simulink model "cart_pend"  (Simulink 7.1)
settings: Solver=ode23  StartTime=0.0  StopTime=5  RelTol=1e-6
values from neighbouring files (symbols this model uses):
  g = 9.81    [MPCsimulink.m]    (also in assignment4.m; pend_init.m; setupOptimization.m)
  g1 = c2d(tf([1 0],[tcAngleVel 1]),h,'tustin')    [assignment4.m]    (also in assignment5.m; pend_init.m)
  g2 = c2d(tf(1,[tcAngle 1]),h,'tustin')    [assignment4.m]    (also in assignment5.m; pend_init.m)
  g3 = c2d(tf(1),h)    [assignment1.m]    (also in assignment3.m = c2d(tf(1,[tcAcc 1]),h,'tustin'); assignment4.m = c2d(tf(1,[tcAcc 1]),h,'tustin'); assignment5.m = c2d(tf(1,[tcAcc 1]),h,'tustin'); pend_init.m = c2d(tf(1,[tcAcc 1]),h,'tustin'))
  h = uIn(5*N+10)    [MPCsimulink.m]    (also in assignment1.m = 0.001; pend_init.m = 0.01)
  initPendValue = [0;0]    [assignment3.m]    (also in assignment4.m; pend_init.m)
  initPosError = 0    [assignment1.m]    (also in assignment3.m; assignment4.m; assignment5.m; pend_init.m)
  l = 0.345    [MPCsimulink.m]    (also in assignment4.m; loaddym.m = fgetl(fid); pend_init.m)
  N = uIn(end)    [MPCsimulink.m]    (also in assignment3.m = -1; assignment5.m = %---------------------------------------------------------; setupOptimization.m = length(theta))
  p0 = -1.5    [assignment1.m]    (also in assignment5.m = -0.8)
  Q = sparse(Q)    [MPCsimulink.m]    (also in assignment3.m = 0; assignment4.m = [  R =; assignment5.m = [  R =)
  R = 0    [assignment3.m]
libraries: simulink x1
settings Model: Creator=pontusg  LastModifiedBy=pontusg  ExtModeAutoUpdateStatusClock=off
settings DataIOCC: Refine=10
settings DebuggingCC: SaveWithParameterizedLinksMsg=none
settings GRTTargetCC: TargetFcnLib=ansi_tfl_tmw.mat

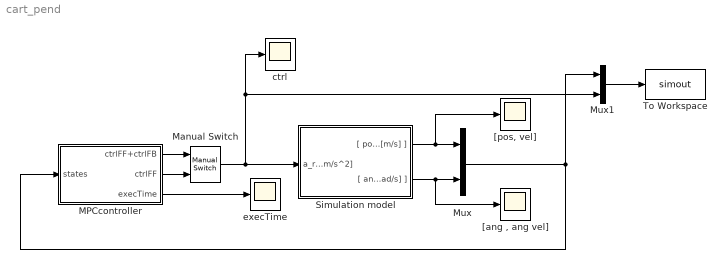
== system cart_pend ==
  MPCcontroller : Subsystem
  Manual Switch : simulink/Signal Routing/Manual Switch  SystemSampleTime=-1  sw=1  action=0  varsize=off
  Mux : Mux  Inputs=2
  Mux1 : Mux  Inputs=2
  Simulation model : Subsystem
  To Workspace : ToWorkspace  VariableName=simout  SampleTime=-1  SaveFormat=Structure With Time
  "[ang , ang vel]" : Scope
      settings: TimeRange=10  YMin=-0.5  YMax=3.25
  "[pos, vel]" : Scope
      settings: TimeRange=6  YMin=-0.0575  YMax=-0.0075
  ctrl : Scope
      settings: TimeRange=10  YMin=-0.5  YMax=3.25  SaveName=ScopeData2
  execTime : Scope
      settings: TimeRange=10  YMin=-0.5  YMax=3.25  SaveName=ScopeData3
  wires:
  Simulation model/1("[ pos [m] , vel [m/s] ]") -> Mux/1, "[pos, vel]"/1
  Mux/1 -> Mux1/1, MPCcontroller/1(states)
  Mux1/1 -> To Workspace/1
  Simulation model/2("[ ang [rad] , angVel [rad/s] ]") -> Mux/2, "[ang , ang vel]"/1
  MPCcontroller/1(ctrlFF+ctrlFB) -> Manual Switch/1
  MPCcontroller/2(ctrlFF) -> Manual Switch/2
  Manual Switch/1 -> ctrl/1, Mux1/2, Simulation model/1(a_ref [m/s^2])
  MPCcontroller/3(execTime) -> execTime/1

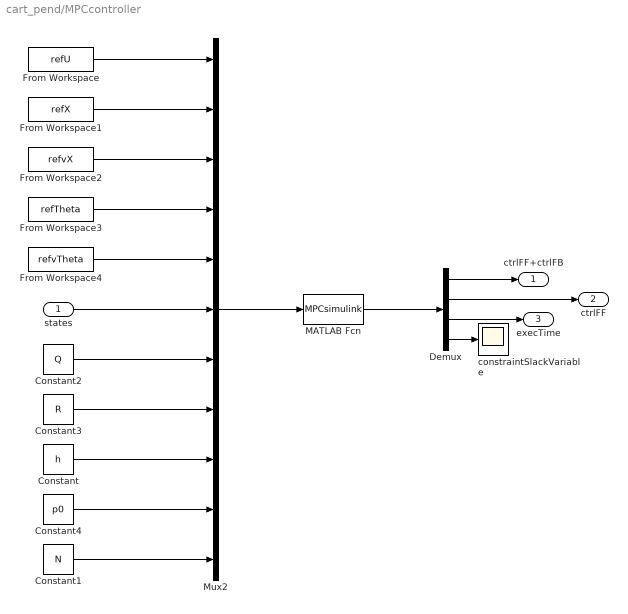
== system cart_pend/MPCcontroller ==
  states : Inport  OutDataType=sfix(16)  OutScaling=2^0
  Constant : Constant  Value=h  OutDataType=sfix(16)  OutScaling=2^0  SampleTime=h
  Constant1 : Constant  Value=N  OutDataType=sfix(16)  OutScaling=2^0  SampleTime=h
  Constant2 : Constant  Value=Q  OutDataType=sfix(16)  OutScaling=2^0  SampleTime=h
  Constant3 : Constant  Value=R  OutDataType=sfix(16)  OutScaling=2^0  SampleTime=h
  Constant4 : Constant  Value=p0  OutDataType=sfix(16)  OutScaling=2^0  SampleTime=h
  Demux : Demux  Outputs=[1 1 1 1]
  From Workspace : FromWorkspace  VariableName=refU  SampleTime=h  Interpolate=off  OutputAfterFinalValue=Holding final value
  From Workspace1 : FromWorkspace  VariableName=refX  SampleTime=h  Interpolate=off  OutputAfterFinalValue=Holding final value
  From Workspace2 : FromWorkspace  VariableName=refvX  SampleTime=h  Interpolate=off  OutputAfterFinalValue=Holding final value
  From Workspace3 : FromWorkspace  VariableName=refTheta  SampleTime=h  Interpolate=off  OutputAfterFinalValue=Holding final value
  From Workspace4 : FromWorkspace  VariableName=refvTheta  SampleTime=h  Interpolate=off  OutputAfterFinalValue=Holding final value
  MATLAB Fcn : MATLABFcn  MATLABFcn=MPCsimulink  OutputDimensions=4
  Mux2 : Mux  Inputs=11
  constraintSlackVariable : Scope
      settings: TimeRange=8.378423004623279  YMin=0.004183789062500001  YMax=0.004352539062500001  SaveName=ScopeData6
  ctrlFF+ctrlFB : Outport  OutDataType=sfix(16)  OutScaling=2^0
  ctrlFF : Outport  Port=2  OutDataType=sfix(16)  OutScaling=2^0
  execTime : Outport  Port=3  OutDataType=sfix(16)  OutScaling=2^0
  wires:
  From Workspace/1 -> Mux2/1
  From Workspace1/1 -> Mux2/2
  From Workspace2/1 -> Mux2/3
  From Workspace3/1 -> Mux2/4
  From Workspace4/1 -> Mux2/5
  Mux2/1 -> MATLAB Fcn/1
  Demux/1 -> ctrlFF+ctrlFB/1
  Demux/2 -> ctrlFF/1
  MATLAB Fcn/1 -> Demux/1
  states/1 -> Mux2/6
  Constant2/1 -> Mux2/7
  Constant3/1 -> Mux2/8
  Constant/1 -> Mux2/9
  Demux/3 -> execTime/1
  Demux/4 -> constraintSlackVariable/1
  Constant4/1 -> Mux2/10
  Constant1/1 -> Mux2/11

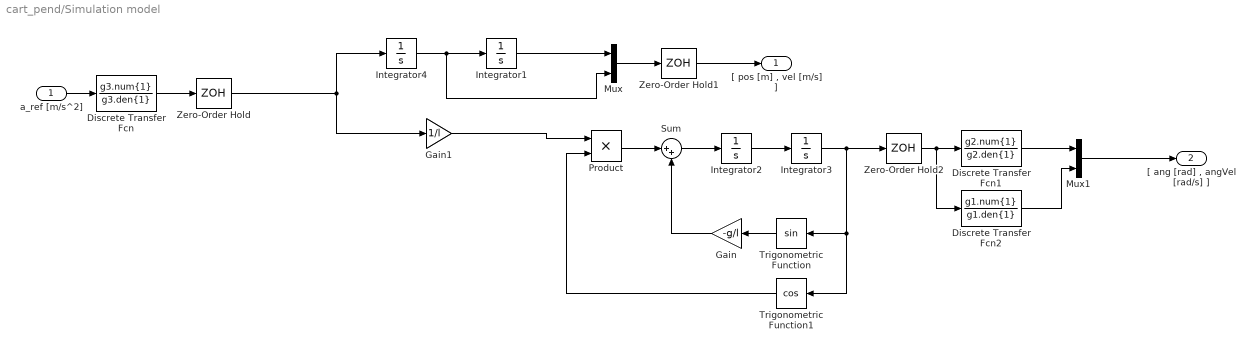
== system cart_pend/Simulation model ==
  a_ref [m/s^2] : Inport  OutDataType=sfix(16)  OutScaling=2^0
  Discrete Transfer Fcn : DiscreteTransferFcn  Numerator=g3.num{1}  Denominator=g3.den{1}  SampleTime=h
  Discrete Transfer Fcn1 : DiscreteTransferFcn  Numerator=g2.num{1}  Denominator=g2.den{1}  SampleTime=h
  Discrete Transfer Fcn2 : DiscreteTransferFcn  Numerator=g1.num{1}  Denominator=g1.den{1}  SampleTime=h
  Gain : Gain  Orientation=left  Gain=-g/l  ParameterDataType=sfix(16)  ParameterScaling=2^0  OutDataType=sfix(16)  OutScaling=2^0
  Gain1 : Gain  Gain=1/l  ParameterDataType=sfix(16)  ParameterScaling=2^0  OutDataType=sfix(16)  OutScaling=2^0
  Integrator1 : Integrator  InitialCondition=p0+initPosError
  Integrator2 : Integrator  InitialCondition=initPendValue(2)
  Integrator3 : Integrator  InitialCondition=initPendValue(1)
  Integrator4 : Integrator
  Mux : Mux  Inputs=2
  Mux1 : Mux  Inputs=2
  Product : Product  OutDataType=sfix(16)  OutScaling=2^0  RndMeth=Zero
  Sum : Sum  Inputs=|++  OutDataType=sfix(16)  OutScaling=2^0
  Trigonometric Function : Trigonometry  Orientation=left
  Trigonometric Function1 : Trigonometry  Orientation=left  Operator=cos
  Zero-Order Hold : ZeroOrderHold  SampleTime=h
  Zero-Order Hold1 : ZeroOrderHold  SampleTime=h
  Zero-Order Hold2 : ZeroOrderHold  SampleTime=h
  "[ pos [m] , vel [m/s] ]" : Outport  OutDataType=sfix(16)  OutScaling=2^0
  "[ ang [rad] , angVel [rad/s] ]" : Outport  Port=2  OutDataType=sfix(16)  OutScaling=2^0
  wires:
  Zero-Order Hold1/1 -> "[ pos [m] , vel [m/s] ]"/1
  Zero-Order Hold/1 -> Gain1/1, Integrator4/1
  Integrator4/1 -> Integrator1/1, Mux/2
  Integrator1/1 -> Mux/1
  Integrator2/1 -> Integrator3/1
  Integrator3/1 -> Trigonometric Function/1, Trigonometric Function1/1, Zero-Order Hold2/1
  Sum/1 -> Integrator2/1
  Mux/1 -> Zero-Order Hold1/1
  Mux1/1 -> "[ ang [rad] , angVel [rad/s] ]"/1
  a_ref [m/s^2]/1 -> Discrete Transfer Fcn/1
  Gain1/1 -> Product/1
  Product/1 -> Sum/1
  Trigonometric Function1/1 -> Product/2
  Trigonometric Function/1 -> Gain/1
  Gain/1 -> Sum/2
  Discrete Transfer Fcn1/1 -> Mux1/1
  Discrete Transfer Fcn2/1 -> Mux1/2
  Zero-Order Hold2/1 -> Discrete Transfer Fcn1/1, Discrete Transfer Fcn2/1
  Discrete Transfer Fcn/1 -> Zero-Order Hold/1
